simulink model "mIO"  (Simulink 8.7)
settings: Solver=ode1  StartTime=0.0  StopTime=inf  FixedStep=Ts  RelTol=1e-3
PostLoadFcn:
  | , if any(exist('dsrtsu_mdlpostloadfcn', 'file') == [2, 3, 6]), try dsrtsu_mdlpostloadfcn('Execute', bdroot); catch fprintf('Error in PostLoadFcn (dsrtsu_mdlpostloadfcn) for model "%s":\n %s\n', bdroot, lasterr); end, end,
InitFcn:
  | param
values from neighbouring files (symbols this model uses):
  dm = 3.8E-6    (= 3.8e-06)    [param.m]    (also in param_2.m)
  eps_dm = 1    [param.m]    (also in param_2.m)
  eps_Jeq = 1    [param.m]    (also in param_2.m)
  Jeq = Jm + (J1+J2)/(n^2)    (= 3.6746e-05)    [param.m]    (also in param_2.m)
  Kemf = 1/(137*2*pi/60)    (= 0.0697028947848)    [param.m]    (also in param_2.m)
  Km = 69.7E-3    (= 0.0697)    [param.m]    (also in param_2.m)
  n = 1    [param.m]    (also in param_2.m)
  R = 112    [param.m]    (also in param_2.m)
  Ts = 1e-2    (= 0.01)    [param.m]    (also in param_2.m = 0.001)
undefined symbols (not defined in the file or in its folder): DiscIntNeverNeededParam, dm_final, Dpos, Dpos_d, Dsp_d, dv, Ipos, Ipos_d, Isp_d, Jeq_final, Npos, Npos_d, Nsp_d, Ppos, Ppos_d, Psp_d, Tc
libraries: rtilib1104 x5
settings Model: DSRTSU_INTERNAL_RTI_VER=450  DSRTSU_INTERNAL_RTI_TYPE=rti1104  DSRTSU_INTERNAL_RTIFPGA=40  Creator=user  LastModifiedBy=diegogm  ExtModeArmWhenConnect=off
settings DataIOCC: SignalLoggingSaveFormat=ModelDataLogs  SaveOutput=off  SignalLoggingName=sigsOut
settings OptimizationCC: BlockReduction=off  ConditionallyExecuteInputs=off  OptimizeBlockIOStorage=off  BufferReuse=off  GlobalBufferReuse=off  ExpressionFolding=off  ExpressionDepthLimit=2147483647  LocalBlockOutputs=off  InitFltsAndDblsToZero=on
settings DebuggingCC: SaveWithParameterizedLinksMsg=none  SignalResolutionControl=TryResolveAllWithWarning  MultiTaskDSMMsg=warning  MultiTaskCondExecSysMsg=none  UnconnectedInputMsg=none  UnconnectedOutputMsg=none  StateNameClashWarn=warning
settings HardwareCC: ProdIntDivRoundTo=Zero  ProdEndianess=BigEndian  ProdHWDeviceType=Generic->Custom  TargetIntDivRoundTo=Zero  TargetEndianess=BigEndian  TargetHWDeviceType=Generic->Custom
settings RTWCC: SystemTargetFile=rti1104.tlc  MakeCommand=make_rti  TemplateMakefile=rti1104.tmf  Description=dSPACE DS1104 Hardware Platform  RetainRTWFile=on
settings STFCustomTargetCC: TargetFcnLib=ansi_tfl_tmw.mat  ParMdlRefBuildCompliant=on  GeneratePreprocessorConditionals=Disable all  SystemTargetFile=rti1104.tlc
settings GRTTargetCC: TargetFcnLib=ansi_tfl_tmw.mat  CompOptLevelCompliant=off  ConcurrentExecutionCompliant=off  CombineOutputUpdateFcns=off  MatFileLogging=off  CPPClassGenCompliant=off  GRTInterface=on  UseToolchainInfoCompliant=off  ExtModeMexFile=noextcomm
settings CustomProperty: DataType=RTWOptions_EnumType_C__Program Files (x86)_dSPACE RCPHIL 2014-B_MATLAB_RTI_RTI1104_TLC_rti1104_1InitialSimState  Value=RUN
settings EnumStrPairs: String=RUN
settings ConfigComp: CovSFcnEnable=off

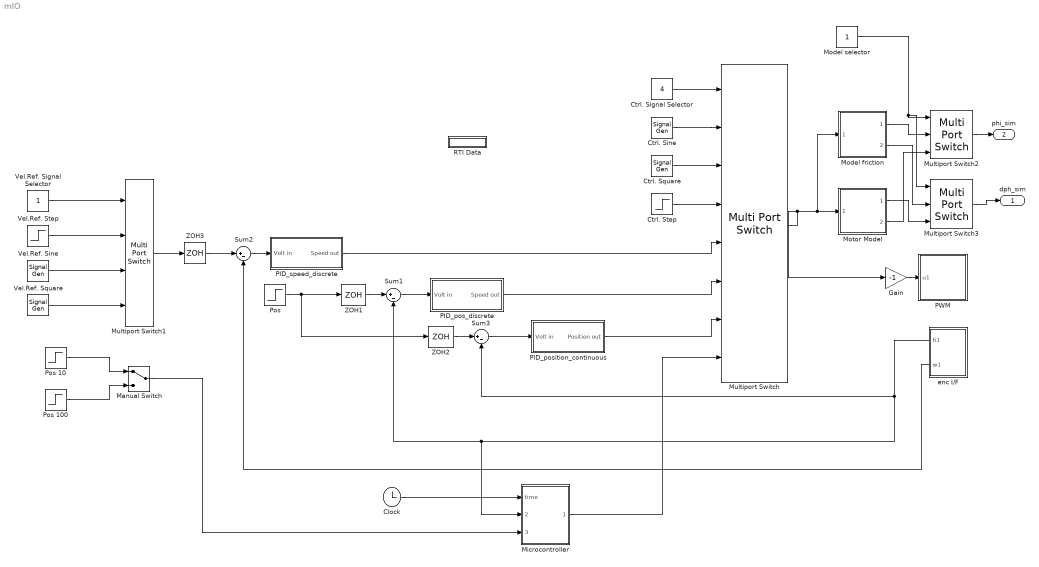
== system mIO ==
  Clock : Clock
  Ctrl. Signal Selector : Constant  Value=4
  Ctrl. Sine : SignalGenerator  Amplitude=24  Frequency=2*pi*2/10  Units=rad/sec
  Ctrl. Square : SignalGenerator  WaveForm=square  Amplitude=24  Frequency=2*pi*2/10  Units=rad/sec
  Ctrl. Step : Step  Time=0  After=24  SampleTime=0
  Gain : Gain  Gain=-1
  Manual Switch : ManualSwitch
  Microcontroller : MATLAB Function  TreatAsAtomicUnit=on  SystemSampleTime=Ts
  "Model friction " : Subsystem
  Model selector : Constant
  Motor Model : Subsystem
  Multiport Switch : MultiPortSwitch  Inputs=7
  Multiport Switch1 : MultiPortSwitch
  Multiport Switch2 : MultiPortSwitch  Inputs=2
  Multiport Switch3 : MultiPortSwitch  Inputs=2
  "PID_pos_discrete  " : Subsystem
  "PID_position_continuous " : Subsystem
  PID_speed_discrete : Subsystem
  PWM : Subsystem
  Pos : Step  Time=0  SampleTime=0
  Pos 10 : Step  Time=0  After=10  SampleTime=0
  Pos 100 : Step  Time=0  After=100  SampleTime=0
  RTI Data : Subsystem  Tag=struct('RTIDataServer',struct('RTIDataServerVs','2','RTIModelDescription','struct(''main'',''mIO'',''sub'','''',''isMp'',0)'))  LoadFcn="if exist('rtidc'), try,  rtidc('DataHostBlockClbLoad', gcbh); catch, disp(['Warning: ''LoadFcn'' for RTI Data block failed: ' lasterr]); end, end,"  mask(RTI_DATA_HOST){}
      mask help:
      | RTI Data Block.
      | This block is used by RTI to store internal model-dependent data.
      | Please keep this block on the root level of the model. Deleting this block will result in data loss.
      |
      | NEVER DELETE OR COPY THIS BLOCK!
      settings: CopyFcn="if exist('rtidc'), try,  rtidc('DataHostBlockClbCopy', gcbh); catch, disp(['Warning: ''CopyFcn'' for RTI Data block failed: ' lasterr]); end, end,"  DeleteFcn="if exist('rtidc'), try,  rtidc('DataHostBlockClbDelete', gcbh); catch, disp(['Warning: ''DeleteFcn'' for RTI Data block failed: ' lasterr]); end, end,"  ModelCloseFcn="if exist('rtidc'), try,  rtidc('DataHostBlockClbModelClose', gcbh); catch, disp(['Warning: ''ModelCloseFcn'' for RTI Data block failed: ' lasterr]); end, end,"  PreSaveFcn="if exist('rtidc'), try,  rtidc('DataHostBlockClbPreSave', gcbh); catch, disp(['Warning: ''PreSaveFcn'' for RTI Data block failed: ' lasterr]); end, end,"  PostSaveFcn="if exist('rtidc'), try,  rtidc('DataHostBlockClbPostSave', gcbh); catch, disp(['Warning: ''PostSaveFcn'' for RTI Data block failed: ' lasterr]); end, end,"  NameChangeFcn="if exist('rtidc'), try,  rtidc('DataHostBlockClbNameChange', gcbh); catch, disp(['Warning: ''NameChangeFcn'' for RTI Data block failed: ' lasterr]); end, end,"
      mask Help:
      | RTI Data Block.
      | This block is used by RTI to store internal model-dependent data.
      | Please keep this block on the root level of the model. Deleting this block will result in data loss.
      | 
      | NEVER DELETE OR COPY THIS BLOCK!
      mask Display:
      | text(0.5, 0.5, 'RTI Data', 'HorizontalAlignment', 'center');
      | plot([1 0]);
  Sum1 : Sum  Inputs=|+-
  Sum2 : Sum  Inputs=|+-
  Sum3 : Sum  Inputs=|+-
  Vel.Ref. Signal Selector : Constant
  Vel.Ref. Sine : SignalGenerator  Amplitude=50  Frequency=2*pi*2/10  Units=rad/sec
  Vel.Ref. Square : SignalGenerator  WaveForm=square  Amplitude=50  Frequency=2/10  Units=rad/sec
  Vel.Ref. Step : Step  Time=0  After=50  SampleTime=0
  ZOH1 : ZeroOrderHold  SampleTime=Ts
  ZOH2 : ZeroOrderHold  SampleTime=Ts
  ZOH3 : ZeroOrderHold  SampleTime=Ts
  enc I/F : Subsystem
  dph_sim : Outport
  phi_sim : Outport  Port=2
  wires:
  Ctrl. Sine/1 -> Multiport Switch/2
  Ctrl. Square/1 -> Multiport Switch/3
  Ctrl. Signal Selector/1 -> Multiport Switch/1
  Ctrl. Step/1 -> Multiport Switch/4
  Gain/1 -> PWM/1(u1)
  Multiport Switch/1 -> Gain/1, "Model friction "/1("Volt in "), Motor Model/1(Signal Input)
  Pos/1 -> ZOH2/1, ZOH1/1
  Sum1/1 -> "PID_pos_discrete  "/1(Volt in)
  Sum3/1 -> "PID_position_continuous "/1(Volt in)
  Sum2/1 -> PID_speed_discrete/1(Volt in)
  ZOH1/1 -> Sum1/1
  "PID_pos_discrete  "/1(Speed out) -> Multiport Switch/6
  ZOH3/1 -> Sum2/1
  PID_speed_discrete/1(Speed out) -> Multiport Switch/5
  ZOH2/1 -> Sum3/1
  enc I/F/2(w1) -> Sum2/2
  enc I/F/1(fi1) -> Sum3/2, Microcontroller/2(Output), Sum1/2
  Multiport Switch1/1 -> ZOH3/1
  Vel.Ref. Step/1 -> Multiport Switch1/2
  Vel.Ref. Signal Selector/1 -> Multiport Switch1/1
  Vel.Ref. Sine/1 -> Multiport Switch1/3
  Vel.Ref. Square/1 -> Multiport Switch1/4
  "PID_position_continuous "/1(Position out) -> Multiport Switch/7
  "Model friction "/1(Pos out) -> Multiport Switch2/2
  Motor Model/2(phi_sim) -> Multiport Switch2/3
  "Model friction "/2(Vel out) -> Multiport Switch3/2
  Multiport Switch2/1 -> phi_sim/1
  Multiport Switch3/1 -> dph_sim/1
  Motor Model/1(dph_sim) -> Multiport Switch3/3
  Model selector/1 -> Multiport Switch3/1, Multiport Switch2/1
  Microcontroller/1(Voltage) -> Multiport Switch/8
  Pos 10/1 -> Manual Switch/1
  Pos 100/1 -> Manual Switch/2
  Manual Switch/1 -> Microcontroller/3(Pos_aim)
  Clock/1 -> Microcontroller/1(time)

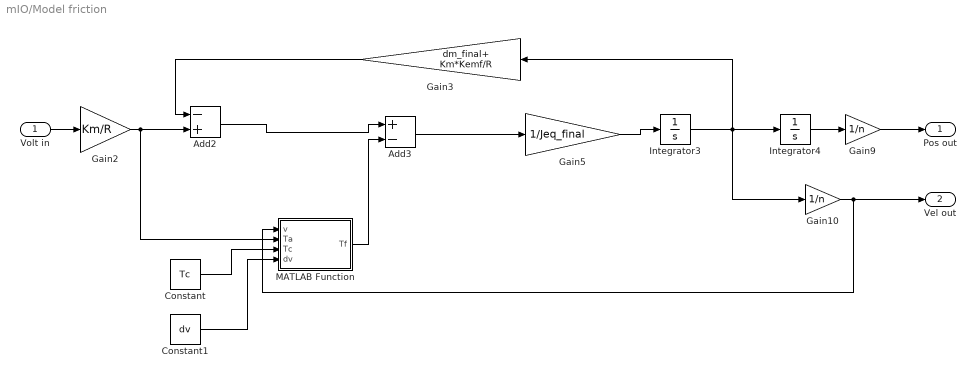
== system mIO/Model friction  ==
  "Volt in " : Inport
  Add2 : Sum  Inputs=-+
  Add3 : Sum  Inputs=+-
  Constant : Constant  Value=Tc
  Constant1 : Constant  Value=dv
  Gain10 : Gain  Gain=1/n
  Gain2 : Gain  Gain=Km/R
  Gain3 : Gain  Gain=dm_final+ Km*Kemf/R
  Gain5 : Gain  Gain=1/Jeq_final
  Gain9 : Gain  Gain=1/n
  Integrator3 : Integrator
  Integrator4 : Integrator
  MATLAB Function : MATLAB Function  TreatAsAtomicUnit=on
  Pos out : Outport
  Vel out : Outport  Port=2
  wires:
  Gain2/1 -> MATLAB Function/2(Ta), Add2/2
  Integrator3/1 -> Integrator4/1, Gain10/1, Gain3/1
  Gain3/1 -> Add2/1
  Gain5/1 -> Integrator3/1
  Integrator4/1 -> Gain9/1
  Gain10/1 -> Vel out/1, MATLAB Function/1(v)
  Add3/1 -> Gain5/1
  Add2/1 -> Add3/1
  MATLAB Function/1(Tf) -> Add3/2
  "Volt in "/1 -> Gain2/1
  Gain9/1 -> Pos out/1
  Constant/1 -> MATLAB Function/3(Tc)
  Constant1/1 -> MATLAB Function/4(dv)

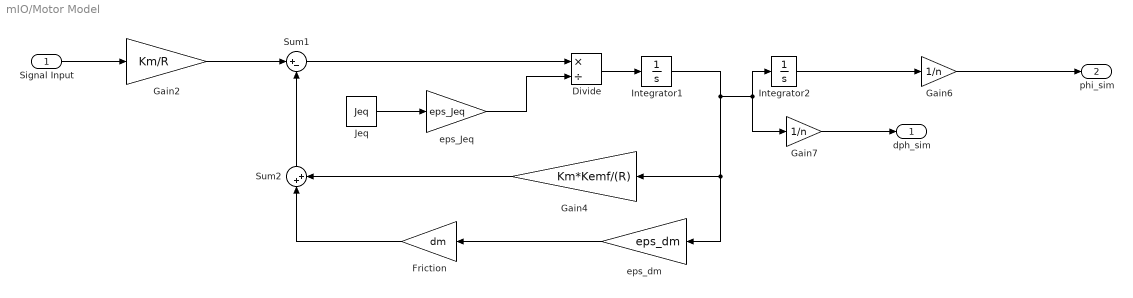
== system mIO/Motor Model ==
  Signal Input : Inport
  Divide : Product  Inputs=*/
  Friction : Gain  Gain=dm
  Gain2 : Gain  Gain=Km/R
  Gain4 : Gain  Gain=Km*Kemf/(R)
  Gain6 : Gain  Gain=1/n
  Gain7 : Gain  Gain=1/n
  Integrator1 : Integrator
  Integrator2 : Integrator
  Jeq : Constant  Value=Jeq
  Sum1 : Sum  Inputs=|+-
  Sum2 : Sum  Inputs=|++
  eps_Jeq : Gain  Gain=eps_Jeq
  eps_dm : Gain  Gain=eps_dm
  dph_sim : Outport
  phi_sim : Outport  Port=2
  wires:
  Integrator1/1 -> eps_dm/1, Gain4/1, Gain7/1, Integrator2/1
  Integrator2/1 -> Gain6/1
  Gain6/1 -> phi_sim/1
  Gain7/1 -> dph_sim/1
  Gain2/1 -> Sum1/1
  Divide/1 -> Integrator1/1
  Friction/1 -> Sum2/1
  Gain4/1 -> Sum2/2
  Sum2/1 -> Sum1/2
  Sum1/1 -> Divide/1
  Jeq/1 -> eps_Jeq/1
  eps_Jeq/1 -> Divide/2
  eps_dm/1 -> Friction/1
  Signal Input/1 -> Gain2/1

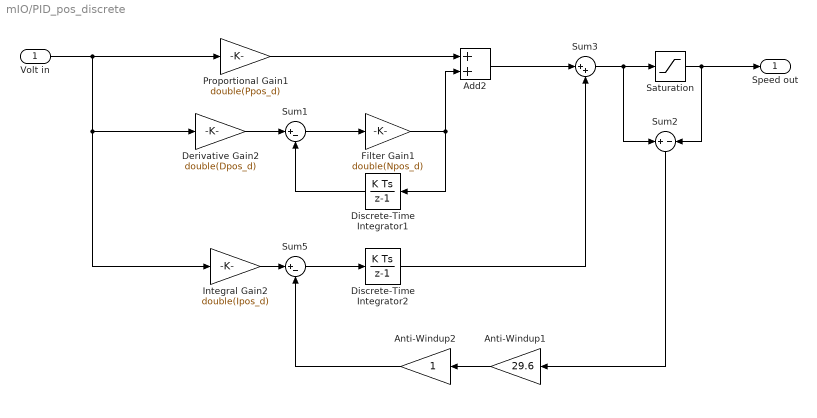
== system mIO/PID_pos_discrete   ==
  Volt in : Inport
  Add2 : Sum
  Anti-Windup1 : Gain  Gain=29.6
  Anti-Windup2 : Gain
  Derivative Gain2 : Gain  Gain=double(Dpos_d)
  Discrete-Time Integrator1 : DiscreteIntegrator  InitialConditionSetting=State (most efficient)  SampleTime=Ts  ICPrevOutput=DiscIntNeverNeededParam  ICPrevScaledInput=DiscIntNeverNeededParam
  Discrete-Time Integrator2 : DiscreteIntegrator  InitialConditionSetting=State (most efficient)  SampleTime=Ts  ICPrevOutput=DiscIntNeverNeededParam  ICPrevScaledInput=DiscIntNeverNeededParam
  Filter Gain1 : Gain  Gain=double(Npos_d)
  Integral Gain2 : Gain  Gain=double(Ipos_d)
  Proportional Gain1 : Gain  Gain=double(Ppos_d)
  Saturation : Saturate  UpperLimit=24  LowerLimit=-24
  Sum1 : Sum  Inputs=|+-
  Sum2 : Sum  Inputs=+|-
  Sum3 : Sum  Inputs=|++
  Sum5 : Sum  Inputs=|+-
  Speed out : Outport
  wires:
  Discrete-Time Integrator2/1 -> Sum3/2
  Add2/1 -> Sum3/1
  Volt in/1 -> Integral Gain2/1, Derivative Gain2/1, Proportional Gain1/1
  Discrete-Time Integrator1/1 -> Sum1/2
  Sum1/1 -> Filter Gain1/1
  Derivative Gain2/1 -> Sum1/1
  Proportional Gain1/1 -> Add2/1
  Filter Gain1/1 -> Discrete-Time Integrator1/1, Add2/2
  Sum3/1 -> Sum2/1, Saturation/1
  Saturation/1 -> Sum2/2, Speed out/1
  Sum2/1 -> Anti-Windup1/1
  Anti-Windup1/1 -> Anti-Windup2/1
  Integral Gain2/1 -> Sum5/1
  Sum5/1 -> Discrete-Time Integrator2/1
  Anti-Windup2/1 -> Sum5/2

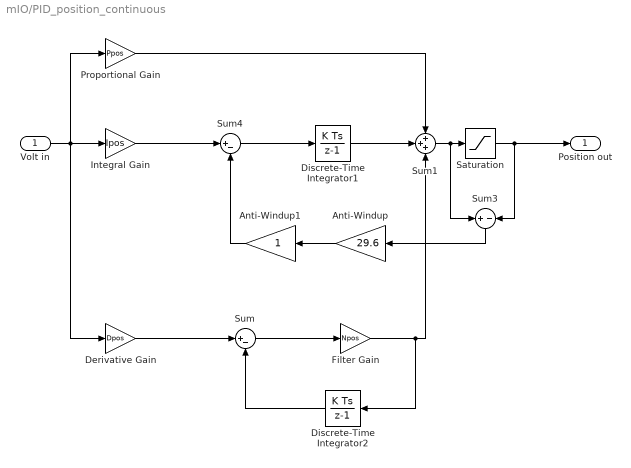
== system mIO/PID_position_continuous  ==
  Volt in : Inport
  Anti-Windup : Gain  Gain=29.6
  Anti-Windup1 : Gain
  Derivative Gain : Gain  Gain=Dpos
  Discrete-Time Integrator1 : DiscreteIntegrator  InitialConditionSetting=State (most efficient)  SampleTime=Ts  ICPrevOutput=DiscIntNeverNeededParam  ICPrevScaledInput=DiscIntNeverNeededParam
  Discrete-Time Integrator2 : DiscreteIntegrator  InitialConditionSetting=State (most efficient)  SampleTime=Ts  ICPrevOutput=DiscIntNeverNeededParam  ICPrevScaledInput=DiscIntNeverNeededParam
  Filter Gain : Gain  Gain=Npos
  Integral Gain : Gain  Gain=Ipos
  Proportional Gain : Gain  Gain=Ppos
  Saturation : Saturate  UpperLimit=24  LowerLimit=-24
  Sum : Sum  Inputs=|+-
  Sum1 : Sum  Inputs=+++
  Sum3 : Sum  Inputs=+|-
  Sum4 : Sum  Inputs=|+-
  Position out : Outport
  wires:
  Discrete-Time Integrator1/1 -> Sum1/2
  Discrete-Time Integrator2/1 -> Sum/2
  Filter Gain/1 -> Discrete-Time Integrator2/1, Sum1/3
  Sum/1 -> Filter Gain/1
  Derivative Gain/1 -> Sum/1
  Proportional Gain/1 -> Sum1/1
  Volt in/1 -> Derivative Gain/1, Integral Gain/1, Proportional Gain/1
  Sum1/1 -> Sum3/1, Saturation/1
  Saturation/1 -> Sum3/2, Position out/1
  Integral Gain/1 -> Sum4/1
  Sum4/1 -> Discrete-Time Integrator1/1
  Sum3/1 -> Anti-Windup/1
  Anti-Windup/1 -> Anti-Windup1/1
  Anti-Windup1/1 -> Sum4/2

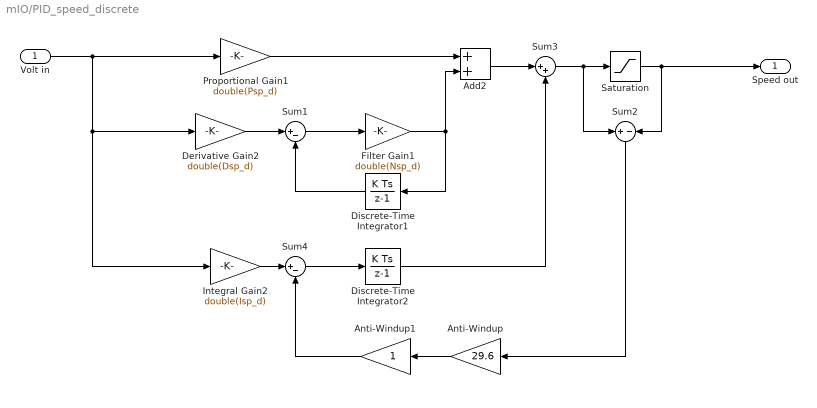
== system mIO/PID_speed_discrete ==
  Volt in : Inport
  Add2 : Sum
  Anti-Windup : Gain  Gain=29.6
  Anti-Windup1 : Gain
  Derivative Gain2 : Gain  Gain=double(Dsp_d)
  Discrete-Time Integrator1 : DiscreteIntegrator  InitialConditionSetting=State (most efficient)  SampleTime=-1  ICPrevOutput=DiscIntNeverNeededParam  ICPrevScaledInput=DiscIntNeverNeededParam
  Discrete-Time Integrator2 : DiscreteIntegrator  InitialConditionSetting=State (most efficient)  SampleTime=-1  ICPrevOutput=DiscIntNeverNeededParam  ICPrevScaledInput=DiscIntNeverNeededParam
  Filter Gain1 : Gain  Gain=double(Nsp_d)
  Integral Gain2 : Gain  Gain=double(Isp_d)
  Proportional Gain1 : Gain  Gain=double(Psp_d)
  Saturation : Saturate  UpperLimit=24  LowerLimit=-24
  Sum1 : Sum  Inputs=|+-
  Sum2 : Sum  Inputs=+|-
  Sum3 : Sum  Inputs=|++
  Sum4 : Sum  Inputs=|+-
  Speed out : Outport
  wires:
  Discrete-Time Integrator2/1 -> Sum3/2
  Add2/1 -> Sum3/1
  Sum3/1 -> Sum2/1, Saturation/1
  Saturation/1 -> Sum2/2, Speed out/1
  Volt in/1 -> Integral Gain2/1, Derivative Gain2/1, Proportional Gain1/1
  Discrete-Time Integrator1/1 -> Sum1/2
  Sum1/1 -> Filter Gain1/1
  Derivative Gain2/1 -> Sum1/1
  Proportional Gain1/1 -> Add2/1
  Filter Gain1/1 -> Discrete-Time Integrator1/1, Add2/2
  Integral Gain2/1 -> Sum4/1
  Sum4/1 -> Discrete-Time Integrator2/1
  Sum2/1 -> Anti-Windup/1
  Anti-Windup/1 -> Anti-Windup1/1
  Anti-Windup1/1 -> Sum4/2

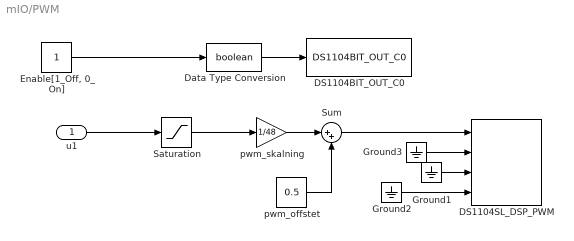
== system mIO/PWM ==
  u1 : Inport
  DS1104BIT_OUT_C0 : rtilib1104/DS1104 MASTER PPC/DS1104BIT_OUT_C0  ChannelNo=0  InitValue=1  TermMode=0  TermValue=0  Reserved1=[]  Reserved2=[]  Reserved3=[]  Reserved=[]  DialogFcn=gui1104bit_out  UnitName={'DS1104BIT_OUT_C'}  UnitValues={ 0 }  DSProperties=struct('RTI',struct('Version',uint32(1),'BlockType',struct('isSLSource',uint8(0),'isSLSink',uint8(1),'isHWSource',uint8(0),'isHWSink',uint8(1),'isSetup',uint8(0),'isInline',uint8(1),'isNonInline',uint8(0),'isInterrupt',uint8(0),'isChannelwise',uint8(1)),'IOBoardType','DS1104MASTER','UnitType','BIT','Identifier','BITOUTCH','DialogType','ML','BlockSet','NONE','SlaveProcessor','NONE'))
  DS1104SL_DSP_PWM : rtilib1104/DS1104 SLAVE DSP/DS1104SL_DSP_PWM  Parameters=[]  TDef=[]  BoardType=[]  PwmMode=1  Frequency=20000  InitValue=[0.5 0.5 0.5 0.5]  TermMode=[0 0 0 0]  TermValue=[0.5 0.5 0.5 0.5]  Polarity=[1 1 1 1]  DialogFcn=gui1104sl_dsp_pwm  Reserved1=[]  Reserved2=[]  Reserved3=[]  Reserved4=[]  Revision=[]  UnitName={'DS1104SL_DSP_PWM'}  UnitValues={[]}  DSProperties=struct('RTI',struct('Version',uint32(2),'BlockType',struct('isSLSource',uint8(0),'isSLSink',uint8(1),'isHWSource',uint8(0),'isHWSink',uint8(1),'isSetup',uint8(0),'isInline',uint8(1),'isNonInline',uint8(0),'isInterrupt',uint8(0),'isChannelwise',uint8(0)),'IOBoardType','DS1104SLAVE','UnitType','PWM','Identifier','PWM','DialogType','ML','BlockSet','NONE','SlaveProcessor','F240'))  RTIBlockInterface=struct('InputPortsActive',[1 1 1 1],'InputPortsWidth',int32([1 1 1 1]),'InputPortsName',{{['PWM Channel 1'],['PWM Channel 2'],['PWM Channel 3'],['PWM Channel 4']}},'IWork',{{{'',uint32(4)}}},'DialogFcn','rti1104slavepwmgui','InitLevel',1,'BlockDisplay',{{'','auto'}},'IconTransparency','on','MultiSFcn',4,'BlockName',struct('Token',{{'DS1104SL_DSP_PWM'}}))  RTIBlockParameters=struct('PWMSymmetryMode',{{1,'OFF',[]}},'PWMFrequency',{{'50000','OFF',[]}},'PWMPolarityMode',{{[1 1 1 1 1],'OFF',[]}},'ChannelNo',{{[1 2 3 4],'OFF',[]}},'SuspendModeInit',{{[0 0 0 0 1],'OFF',[]}},'TTLModeInit',{{[2 2 2 2 2],'OFF',[]}},'DutyCycleInitValueCh1',{{'0.5','OFF',[]}},'DutyCycleInitValueCh2',{{'0.5','OFF',[]}},'DutyCycleInitValueCh3',{{'0.5','OFF',[]}},'DutyCycleInitValueCh4',{{'0.5','OFF',[]}},'DutyCycleInitValueCh5',{{'0.5','OFF',[]}},'EnablePWMStop',{{[0 0 0 0 0],'OFF',[]}},'SuspendModeTerm',{{[0 0 0 0 1],'OFF',[]}},'TTLModeTerm',{{[2 2 2 2 2],'OFF',[]}},'DutyCycleTermValueCh1',{{'0.5','OFF',[]}},'DutyCycleTermValueCh2',{{'0.5','OFF',[]}},'DutyCycleTermValueCh3',{{'0.5','OFF',[]}},'DutyCycleTermValueCh4',{{'0.5','OFF',[]}},'DutyCycleTermValueCh5',{{'0.5','OFF',[]}},'TLCFileName',{{'rti1104pwm','OFF',[]}})  RTISFcnParameters=struct('PWMSymmetryMode','double','PWMFrequency','double','PWMPolarityMode','double','ChannelNo','double','SuspendModeInit','double','TTLModeInit','double','DutyCycleInitValueCh1','double','DutyCycleInitValueCh2','double','DutyCycleInitValueCh3','double','DutyCycleInitValueCh4','double','EnablePWMStop','double','SuspendModeTerm','double','TTLModeTerm','double','DutyCycleTermValueCh1','double','DutyCycleTermValueCh2','double','DutyCycleTermValueCh3','double','DutyCycleTermValueCh4','double','TLCFileName','char')  RTIBlockParaDefault=struct('PWMSymmetryMode',1,'PWMFrequency',100,'PWMPolarityMode',[1 1 1 1 1],'ChannelNo',[1 2 3 4],'SuspendModeInit',[1 1 1 1 1],'TTLModeInit',[2 2 2 2 2],'DutyCycleInitValueCh1',0.5,'DutyCycleInitValueCh2',0.5,'DutyCycleInitValueCh3',0.5,'DutyCycleInitValueCh4',0.5,'DutyCycleInitValueCh5',0.5,'EnablePWMStop',[1 1 1 1 0],'SuspendModeTerm',[1 1 1 1 1],'TTLModeTerm',[2 2 2 2 2],'DutyCycleTermValueCh1',0.5,'DutyCycleTermValueCh2',0.5,'DutyCycleTermValueCh3',0.5,'DutyCycleTermValueCh4',0.5,'DutyCycleTermValueCh5',0.5,'TLCFileName','rti1104pwm')
  Data Type Conversion : DataTypeConversion  OutDataTypeStr=boolean  SaturateOnIntegerOverflow=on  RndMeth=Zero
  "Enable[1_Off, 0_On]" : Constant
  Ground1 : Ground
  Ground2 : Ground
  Ground3 : Ground
  Saturation : Saturate  UpperLimit=24  LowerLimit=-24
  Sum : Sum  Inputs=|++  SaturateOnIntegerOverflow=on
  pwm_offstet : Constant  Value=0.5
  pwm_skalning : Gain  Gain=1/48  SaturateOnIntegerOverflow=on  OutDataTypeStr=Inherit: Same as input  ParamDataTypeStr=Inherit: Same as input
  wires:
  "Enable[1_Off, 0_On]"/1 -> Data Type Conversion/1
  Data Type Conversion/1 -> DS1104BIT_OUT_C0/1
  pwm_skalning/1 -> Sum/1
  Sum/1 -> DS1104SL_DSP_PWM/1
  pwm_offstet/1 -> Sum/2
  u1/1 -> Saturation/1
  Ground1/1 -> DS1104SL_DSP_PWM/3
  Ground2/1 -> DS1104SL_DSP_PWM/4
  Ground3/1 -> DS1104SL_DSP_PWM/2
  Saturation/1 -> pwm_skalning/1

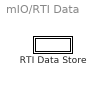
== system mIO/RTI Data ==
  RTI Data Store : Subsystem  Tag="struct('public',struct('sub',struct('name',{{'mIO'}},'data',{{struct('TH',struct('thTaskInfo',struct('taskType',{'TIMER','HWINT','TMRINT','SWINT','GLINT'},'tasksNumOf',{1,0,0,0,0},'srcIds',{{'TIMERA'},{},{},{},{}},'taskNames',{{['Timer Task 1']},{},{},{},{}})),'th_tc',struct('dataType','TASK','taskGroupId','','taskGroupList',{{}},'taskSchedulingPolicy','FCFS','taskType','TIMER','blkh',-1,'srcId','TIMERA','srcSgnName',['Timer A interrupt'],'srcCpuName','','taskName',['Timer Task 1  [0.025] s'],'taskNameDisplayExt','','smplTime',0.025,'smplTimeOffs',0,'hasFixedPriority',0,'priority',1,'hasFixedOvc',0,'ovcType',1,'ovcMax',1),'tc_th',struct('dataType','TASK','taskGroupId','','taskGroupList',{{}},'taskSchedulingPolicy','FCFS','taskType','TIMER','blkh',-1,'srcId','TIMERA','srcSgnName',['Timer A interrupt'],'srcCpuName','','taskName',['Timer Task 1  [0.025] s'],'taskNameDisplayExt','','smplTime',0.025,'smplTimeOffs',0,'hasFixedPriority',0,'priority',1,'hasFixedOvc',0,'ovcType',1,'ovcMax',1))}})),'private',struct('version',struct('dsVer',uint32(2)),'access',struct('modified',['27-Mar-2017 14:18:22'],'type','Model','isPerm',1)))"  mask(RTI_DATA_STORE){}
      mask help:
      | RTI Data Store Block. This block is used by RTI to store internal model dependent data. Deleting this block will result in data loss.
      |
      | NEVER DELETE, COPY, OR MODIFY THIS BLOCK!
      mask Help:
      | RTI Data Store Block. This block is used by RTI to store internal model dependent data. Deleting this block will result in data loss.
      | 
      | NEVER DELETE, COPY, OR MODIFY THIS BLOCK!
      mask Display: text(0.5, 0.5, ' ', 'HorizontalAlignment', 'center');

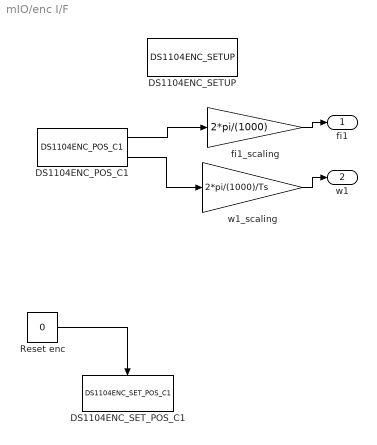
== system mIO/enc I/F ==
  DS1104ENC_POS_C1 : rtilib1104/DS1104 MASTER PPC/DS1104ENC_POS_C1  ChannelNo=1  PosValue=0  Reserved1=[]  Reserved2=[]  Reserved3=[]  Reserved4=[]  DialogFcn=gui1104enc_pos  UnitName={'DS1104ENC_POS_C'}  UnitValues={ 1 }  DSProperties=struct('RTI',struct('Version',uint32(1),'BlockType',struct('isSLSource',uint8(1),'isSLSink',uint8(0),'isHWSource',uint8(1),'isHWSink',uint8(0),'isSetup',uint8(0),'isInline',uint8(1),'isNonInline',uint8(0),'isInterrupt',uint8(0),'isChannelwise',uint8(1)),'IOBoardType','DS1104MASTER','UnitType','ENC','Identifier','ENCPOSCH','DialogType','ML','BlockSet','NONE','SlaveProcessor','NONE'))
  DS1104ENC_SETUP : rtilib1104/DS1104 MASTER PPC/DS1104ENC_SETUP  Reserved1=[]  Reserved2=[]  Reserved3=[]  Reserved4=[]  DialogFcn=gui1104enc_setup  UnitName={'DS1104ENC_SETUP'}  UnitValues={ [] }  DSProperties=struct('RTI',struct('Version',uint32(1),'BlockType',struct('isSLSource',uint8(0),'isSLSink',uint8(0),'isHWSource',uint8(0),'isHWSink',uint8(0),'isSetup',uint8(0),'isInline',uint8(1),'isNonInline',uint8(0),'isInterrupt',uint8(0),'isChannelwise',uint8(0)),'IOBoardType','DS1104MASTER','UnitType','ENC','Identifier','ENCSETUP','DialogType','ML','BlockSet','NONE','SlaveProcessor','NONE'))
      settings: SignalType=[1 0]
  DS1104ENC_SET_POS_C1 : rtilib1104/DS1104 MASTER PPC/DS1104ENC_SET_POS_C1  ChannelNo=1  PosValue=0  Reserved1=[]  Reserved2=[]  Reserved3=[]  Reserved4=[]  DialogFcn=gui1104enc_set_pos  UnitName={'DS1104ENC_SET_POS_C'}  UnitValues={ 1 }  DSProperties=struct('RTI',struct('Version',uint32(1),'BlockType',struct('isSLSource',uint8(0),'isSLSink',uint8(1),'isHWSource',uint8(0),'isHWSink',uint8(1),'isSetup',uint8(0),'isInline',uint8(1),'isNonInline',uint8(0),'isInterrupt',uint8(0),'isChannelwise',uint8(1)),'IOBoardType','DS1104MASTER','UnitType','ENC','Identifier','ENCRESET','DialogType','ML','BlockSet','NONE','SlaveProcessor','NONE'))
  Reset enc : Constant  Value=0
  fi1_scaling : Gain  Gain=2*pi/(1000)  SaturateOnIntegerOverflow=on  OutDataTypeStr=Inherit: Same as input  ParamDataTypeStr=Inherit: Same as input
  w1_scaling : Gain  Gain=2*pi/(1000)/Ts  SaturateOnIntegerOverflow=on  OutDataTypeStr=Inherit: Same as input  ParamDataTypeStr=Inherit: Same as input
  fi1 : Outport
  w1 : Outport  Port=2
  wires:
  Reset enc/1 -> DS1104ENC_SET_POS_C1/Trigger
  DS1104ENC_POS_C1/1 -> fi1_scaling/1
  DS1104ENC_POS_C1/2 -> w1_scaling/1
  fi1_scaling/1 -> fi1/1
  w1_scaling/1 -> w1/1

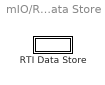
== system mIO/RTI Data/RTI Data Store ==
  RTI Data Store : Subsystem  mask(RTI_DATA_STORE){}
      mask help:
      | RTI Data Store Block. This block is used by RTI to store internal model dependent data. Deleting this block will result in data loss.
      |
      | NEVER DELETE, COPY, OR MODIFY THIS BLOCK!
      mask Help:
      | RTI Data Store Block. This block is used by RTI to store internal model dependent data. Deleting this block will result in data loss.
      | 
      | NEVER DELETE, COPY, OR MODIFY THIS BLOCK!
      mask Display: text(0.5, 0.5, ' ', 'HorizontalAlignment', 'center');

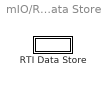
== system mIO/RTI Data/RTI Data Store/RTI Data Store ==
  RTI Data Store : Subsystem  mask(RTI_DATA_STORE){}
      mask help:
      | RTI Data Store Block. This block is used by RTI to store internal model dependent data. Deleting this block will result in data loss.
      |
      | NEVER DELETE, COPY, OR MODIFY THIS BLOCK!
      mask Help:
      | RTI Data Store Block. This block is used by RTI to store internal model dependent data. Deleting this block will result in data loss.
      | 
      | NEVER DELETE, COPY, OR MODIFY THIS BLOCK!
      mask Display: text(0.5, 0.5, ' ', 'HorizontalAlignment', 'center');

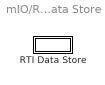
== system mIO/RTI Data/RTI Data Store/RTI Data Store/RTI Data Store ==
  RTI Data Store : Subsystem  mask(RTI_DATA_STORE){}
      mask help:
      | RTI Data Store Block. This block is used by RTI to store internal model dependent data. Deleting this block will result in data loss.
      |
      | NEVER DELETE, COPY, OR MODIFY THIS BLOCK!
      mask Help:
      | RTI Data Store Block. This block is used by RTI to store internal model dependent data. Deleting this block will result in data loss.
      | 
      | NEVER DELETE, COPY, OR MODIFY THIS BLOCK!
      mask Display: text(0.5, 0.5, ' ', 'HorizontalAlignment', 'center');

== system mIO/RTI Data/RTI Data Store/RTI Data Store/RTI Data Store/RTI Data Store ==

== matlab function Microcontroller ==
  data: time input double; Output input double; Pos_aim input double; Voltage output double
function Voltage   = Planner(time,Output, Pos_aim)
    
    %%%%%%%%%%%%%%%%%%%%%%%%%
    %%Parameter declaration%%
    %%%%%%%%%%%%%%%%%%%%%%%%%

    R = 112;
    Km = 69.7E-3;
    Kemf = 1/(137*2*pi/60);
    dm = 3.8E-6;
    Jm = 7.46/(1000*100^2);
    J1 = 1.8E-5;
    J2 = 1.8E-5;
    n = 1;
    Jeq = Jm + (J1+J2)/(n^2);
    %Calculated parameters for the DC motor used in the workshops
    eps_Jeq = 0.6; % Scaling factor for inertia
    eps_dm = 3.56; % scaling blabals
    
    Jeq = eps_Jeq*Jeq;
    dm = dm*eps_dm; 
    %Coulomb friction
    Fc = 0.0013;
    
    %Sampling time
    Ts = 5e-3;
    %%%%%%%%%%%%%%%%%%%%%%%%%%%%%%%%%%%%%%%%%%
    %%Trayectory planner - Signal generation%%
    %%%%%%%%%%%%%%%%%%%%%%%%%%%%%%%%%%%%%%%%%%
    
    %Define a rising time. The motor will be accelerating during 0.5 s.
    %Then it will have 0 acceleration over 0.5 s. Last step would be that
    %it accelerate in the opposite direction for 0.5 s. This acceleration
    %will be one such that it will never pass the maximum acceleration
    %(calculated in the following lines) and that ensures that the final
    %position is the one desired. 
    
    %Motor characteristics - from datasheet. We use a margin of 20% as the
    %PID controller will need some margins for operate correctly. 
    MaxCurrent = 0.182*0.8;
    MaxVoltage = 24*0.8;
    
    %Max dynamics
    Max_Speed_ref = MaxVoltage/Kemf;
    Max_Accel_ref = Km*MaxCurrent/Jeq;
    
    %Definition of trising
    trising = 0.5;
    
    %We calculate the speed and acceleration that we need to get to the
    %position given the trising time. 
    Max_Speed = Pos_aim/(2*trising);
    Max_Accel = Max_Speed/trising;
    
    %Check that we are inside the Max_acceleration and Max_speed boundaries
    if Max_Speed > Max_Speed_ref || Max_Accel > Max_Accel_ref
        disp('Error, Speed/Accel too high')
        pause();
    end 
    
    %Definition of the time that the motor will have 0 acceleration
    t_est = (Pos_aim - Max_Speed*trising)/Max_Speed;
    
    %If we haven't reached the trising time, the motor accelerates
    if time < trising
        signal_accel = Max_Accel;
    %If we reach this values, and have not reached t_est time, the motor
    %has 0 acceleration
    elseif time >= trising && time < (trising + t_est)
        signal_accel = 0; 
    %If we pass t_est, then it accelerates again but inversely
    elseif time >= (trising + t_est) && time < (2*trising + t_est)
        signal_accel = - Max_Accel;
    %when it has accelerated during trising, the acceleration remains
    %steady in 0.
    else
        signal_accel = 0;
    end
    
    %%%%%%%%%%%%%%%%%%%%%%%%%%%%%%%%%%%%%%%%%%%%%%%%%
    %%Trayectory planner - Acceleration integration%%
    %%%%%%%%%%%%%%%%%%%%%%%%%%%%%%%%%%%%%%%%%%%%%%%%%
    
    %We need to integrate the acceleration: once to get the velocity and
    %twice to get the position. This is done, in the discrete time: 
    %
    %   - Speed = (Ts/(z-1))*Accel
    %   - Pos = (Ts/(z-1))*Speed
    %
    %Translated this to code-style language, we have: 
    %
    %   - Speed(n) = Ts*Accel(n) + Speed(n-1)
    %   - Pos(n) = Ts*Speed(n) + Pos(n-1)
    
    %We need to store values from previous calls of this function, then: 
    %Declaration of Speed(n_1)
    persistent outspeed_n_1;
    %Declaration of Pos(n_1)
    persistent outpos_n_1;
    
    %Initialization to 0 of these variables
    if isempty(outspeed_n_1)
        outspeed_n_1 = 0;
    end
    if isempty(outpos_n_1)
        outpos_n_1 = 0;
    end
    
    %The acceleration is not changed, we just need it to calculate the
    %Speed and the postion.
    Speed = signal_accel*Ts + outspeed_n_1;
    outspeed_n_1 = Speed;
    Position = Speed*Ts + outpos_n_1;
    outpos_n_1 = Position;
    
    %%%%%%%%%%%%%%%%%%%%%%%%%%%%%%%%%
    %%Model planner - inverse model%%
    %%%%%%%%%%%%%%%%%%%%%%%%%%%%%%%%%
    
    % We inverse the motor model to get the voltage we need to get a
    % certain acceleration and voltage.  
    Voltage_Planner = (Speed*dm + signal_accel*Jeq + sign(Speed)*Fc)*R/Km + Km*Speed; 
    
    %%%%%%%%%%%%%%%%%%%%
    %%PID - controller%%
    %%%%%%%%%%%%%%%%%%%%
    %
    %We calculated a PID controller for the DC motor model using Pole
    %Placement, implemented as a matlab function for both workshops A and
    %B. We did not need a fast-response controller. The controller we
    %designed is: 
    %
    %         758.5 z^2 - 1393 z + 640.5
    %   PID = ---------------------------
    %          z^2 - 0.9268 z - 0.07323
    %
    %Rewriting this in a code-style, we get: 
    %
    %Out(n) = In(n)*758.5 + In(n-1)*(-1393) + In(n-2)*640.5 - Out(n-1)*(-0.9268) - Out(n-2)*(-0.07323);
    
    %We need again to declare some variables as persistent, as they have to
    %be used in different iterations of the function
    persistent Out_n_1;
    persistent Out_n_2;
    persistent In_n_1;
    persistent In_n_2;
    
    %Initialization of persistent variables
    if isempty(Out_n_1)
        Out_n_1 = 0;
    end
    if isempty(Out_n_2)
        Out_n_2 = 0;
    end
    if isempty(In_n_1)
        In_n_1 = 0;
    end
    if isempty(In_n_2)
        In_n_2 = 0;
    end
    
    %Declaration of the parameters of the PID
    PID_den = [1 -0.9268 -0.07323];
    PID_num = [758.5 -1393 640.5];
    
    %Is an error PID so we need to substract the actual position from the
    %aimed position. 
    Error = Position - Output; 
    
    %Main PID function
    Voltage_Controller = Error*PID_num(1) + In_n_1*PID_num(2) + In_n_2*PID_num(3) - Out_n_1*PID_den(2) - Out_n_2*PID_den(3);
    
    %Store the values for next iterations
    In_n_2 = In_n_1;
    In_n_1 = Error;
    Out_n_2 = Out_n_1;
    Out_n_1 = Voltage_Controller;
    
    %The last step will be to add both voltages, from the controller and
    %the trayectory planner
    Voltage = Voltage_Controller + Voltage_Planner;
end

== matlab function Model friction /MATLAB Function ==
  data: v input double; Tf output double; Ta input double; Tc input double; dv input double
function Tf = fcn(v,Ta,Tc,dv)

if abs(v) < dv
    if abs(Ta) > Tc
        Tf = Tc*sign(Ta);
    else
        Tf = Ta;
    end
else
    Tf = Tc*sign(v);
end
